simulink model "PID_CTRL"  (R2020b)
settings: Solver=VariableStepAuto  StartTime=0.0  StopTime=10.0  RelTol=1e-3
model workspace (MAT data in the model file):
  Kd = Simulink.Parameter
  Kd.Value = 346
  Kd.DataType = 'auto'
  Kd.Dimensions = [1 1]
  Ki = Simulink.Parameter
  Ki.Value = 76
  Ki.DataType = 'auto'
  Ki.Dimensions = [1 1]
  Kp = Simulink.Parameter
  Kp.Value = 1000
  Kp.DataType = 'auto'
  Kp.Dimensions = [1 1]
values from neighbouring files (symbols this model uses):
  Kd = 346    [parameters.m]
  Ki = 76    [parameters.m]
  Kp = 1000    [parameters.m]
settings Model: DataDictionary=cruise.sldd  Creator=sushma  LastModifiedBy=sushma
settings DataIOCC: SaveOutput=off  SaveTime=off

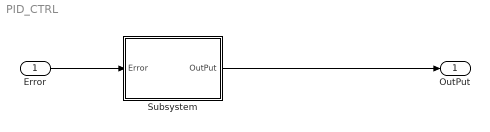
== system PID_CTRL ==
  Error : Inport  OutDataTypeStr=double  PortDimensions=1  SampleTime=0
  Subsystem : Subsystem  TreatAsAtomicUnit=on
  OutPut : Outport  OutDataTypeStr=double  PortDimensions=1  SampleTime=0
  wires:
  Error/1 -> Subsystem/1(Error)
  Subsystem/1(OutPut) -> OutPut/1

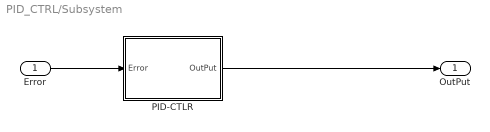
== system PID_CTRL/Subsystem ==
  Error : Inport
  PID-CTLR : Subsystem
  OutPut : Outport
  wires:
  Error/1 -> PID-CTLR/1(Error)
  PID-CTLR/1(OutPut) -> OutPut/1

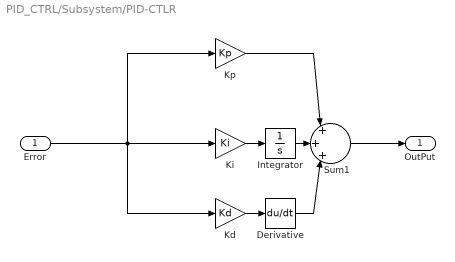
== system PID_CTRL/Subsystem/PID-CTLR ==
  Error : Inport  OutDataTypeStr=double  PortDimensions=1
  Derivative : Derivative
  Integrator : Integrator
  Kd : Gain  Gain=Kd
  Ki : Gain  Gain=Ki
  Kp : Gain  Gain=Kp
  Sum1 : Sum  Inputs=|+|+|+|
  OutPut : Outport  OutDataTypeStr=double  PortDimensions=1  SampleTime=0
  wires:
  Sum1/1 -> OutPut/1
  Kp/1 -> Sum1/1
  Derivative/1 -> Sum1/3
  Integrator/1 -> Sum1/2
  Ki/1 -> Integrator/1
  Error/1 -> Kd/1, Kp/1, Ki/1
  Kd/1 -> Derivative/1
